simulink model "model2"  (R2023a)
settings: Solver=ode45  StartTime=0.0  StopTime=6  FixedStep=dt  MaxStep=0.001  RelTol=1e-3
values from neighbouring files (symbols this model uses):
  A = simplify(A)    [controllabilityLevel_btw.m]    (also in linearizationSS_syms.m = subs(nabla_fVec_x, args_vec, S0))
  B = simplify(B)    [controllabilityLevel_btw.m]    (also in linearizationSS_syms.m = subs(nabla_fVec_u, args_vec, S0))
  C = subs(nabla_hVec_x, args_vec, S0)    [linearizationSS_syms.m]    (also in main1_finHorLQR_OperatingPoint.m = eye(4,4); main2_finHorLQR_program_Trajectory.m = eye(4,4))
  D = subs(nabla_hVec_u, args_vec, S0)    [linearizationSS_syms.m]    (also in main1_finHorLQR_OperatingPoint.m = zeros(4,1); main2_finHorLQR_program_Trajectory.m = zeros(4,1))
  enableLinmodel = 0    [ALLINONE.m]    (also in main1_finHorLQR_OperatingPoint.m = 1; main2_finHorLQR_program_Trajectory.m)
  IC = [track_len/2, pi, 0, 0]'    [ALLINONE.m]    (also in main1_finHorLQR_OperatingPoint.m = [track_len/2;the0deg*pi/180;0;0]; main2_finHorLQR_program_Trajectory.m = [track_len/2;the0deg*pi/180;0;0])
  sat = [12, -12]    [ALLINONE.m]    (also in main1_finHorLQR_OperatingPoint.m; main2_finHorLQR_program_Trajectory.m)
settings Model: Creator=Adam  LastModifiedBy=domrazek
settings SolverCC: AlgebraicLoopSolver=TrustRegion
settings DataIOCC: ExternalInput=ind  LoadExternalInput=on  SignalLogging=off  DSMLogging=off  OutputSaveName=out  ReturnWorkspaceOutputsName=sout
settings OptimizationCC: SimCompilerOptimization=on  AccelVerboseBuild=on
settings DebuggingCC: AlgebraicLoopMsg=none  UnconnectedInputMsg=warning  UnconnectedOutputMsg=warning  UnconnectedLineMsg=warning
settings ModelReferenceCC: EnableRefExpFcnMdlSchedulingChecks=on
settings RTWCC: DLArmComputeVersion=19.05

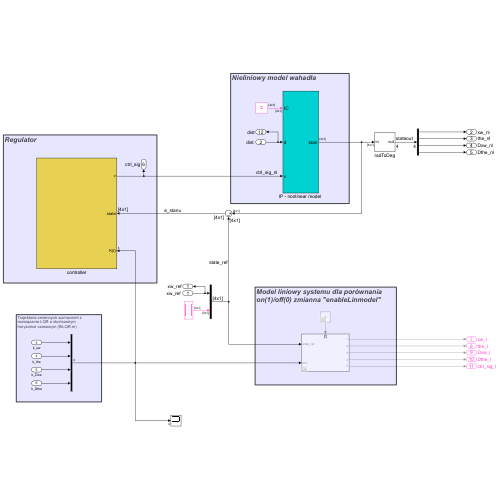
[thumbnail: Simulink's stored preview of the top-level diagram]
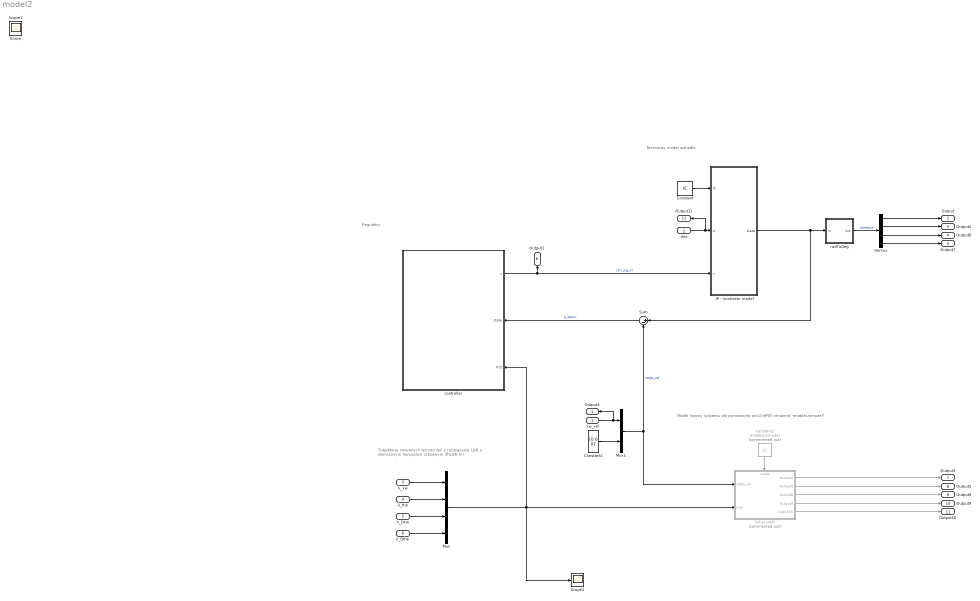
== system model2 ==
  note: Trajektoria zmiennych wzmocnień z
      | rozwiązania LQR o skończonym
      | horyzońce czasowym (fhLQR.m)
  note: Model liniowy systemu dla porównania
      | on(1)/off(0) zmianna "enableLinmodel"
  note: Nieliniowy model wahadła
  note: Regulator
  xw_ref : Inport
  dist : Inport  Port=2
  k_xw : Inport  Port=3
  k_the : Inport  Port=4
  k_Dxw : Inport  Port=5
  k_Dthe : Inport  Port=6
  Constant : Constant  Value=IC  VectorParams1D=off
  Constant1 : Constant  Value=[0 0 0]'  VectorParams1D=off
  Constant2 : Constant  Commented=on  Value=enableLinmodel
  Demux : Demux
  "IP - nonlinear model " : Subsystem  Description=Nonlinear model of inverted pendulum
      mask Display:
      | port_label('output', 1, 'stan');
      | port_label('input', 1, 'IC');
      | port_label('input', 2, 'd');
      | port_label('input', 3, 'v');
  Mux : Mux
  Mux1 : Mux  Inputs=2
  Scope2 : Scope
  Subsystem : Subsystem  Commented=on
  Sum : Sum  Inputs=|+-
  controller : Subsystem
      settings: PortSchema="{\"entries\":[{\"content\":{\"sides\":[{\"content\":{},\"type\":\"ConnectorPlacement.EquallySpacedRectSide\",\"uuid\":\"6de1dc69-5efb-4201-9eee-dce886879f47\"},{\"content\":{\"connectorIds\":[\"Out1\",\"In1\",\"In2\"],\"side\":\"RIGHT\"},\"type\":\"ConnectorPlacement.EquallySpacedRectSide\",\"uuid\":\"f5fecc05-d223-4a83-8c79-e750f1bc671b\"},{\"content\":{\"side\":\"TOP\"},\"type\":\"ConnectorPlacement.EquallySpacedRectSide\",\"uuid\":\"1fb1d94d-6570-44f6-b110-6f3978b46153\"},{\"content\":{\"side\":\"BOTTOM\"},\"type\":\"ConnectorPlacement.EquallySpacedRectSide\",\"uuid\":\"9cfdfd1f-f92b-46ce-ad17-e53ae881dd94\"}]},\"type\":\"ConnectorPlacement.EquallySpacedConnector\",\"uuid\":\"82464fa0-0bcf-47e2-bfa0-6457bd20ad21\"}],\"packageUris\":[\"http://schema.mathworks.com/mf0/Connector/R2020b\"],\"version\":\"1.0\"}"
  radToDeg : Subsystem
  Output4 : Outport  SignalName=xw_ref
  Output : Outport  Port=2  SignalName=xw_nl
  Output2 : Outport  Port=3  SignalName=the_nl
  Output6 : Outport  Port=4  SignalName=Dxw_nl
  Output7 : Outport  Port=5  SignalName=Dthe_nl
  Output1 : Outport  Port=6  SignalName=ctrl_sig
  Output3 : Outport  Port=7  SignalName=xw_l
  Output5 : Outport  Port=8  SignalName=the_l
  Output8 : Outport  Port=9  SignalName=Dxw_l
  Output9 : Outport  Port=10  SignalName=Dthe_l
  Output10 : Outport  Port=11  SignalName=ctrl_sig_l
  Output11 : Outport  Port=12  SignalName=dist
  Scope : Scope
  Scope1 : Scope
  wires:
  "IP - nonlinear model "/1(state) -> radToDeg/1(in), Sum/1
  Constant/1 -> "IP - nonlinear model "/1(IC)
  controller/1(v) -> Output1/1, "IP - nonlinear model "/3(v)  "ctrl_sig_nl"
  Sum/1 -> controller/1(state)  "e_stanu"
  dist/1 -> Output11/1, "IP - nonlinear model "/2(d)
  radToDeg/1(out) -> Demux/1  "stateout"
  Constant1/1 -> Mux1/2
  xw_ref/1 -> Output4/1, Mux1/1
  Mux1/1 -> Subsystem/1(state_ref), Sum/2  "state_ref"
  Demux/1 -> Output/1
  Demux/2 -> Output2/1
  Demux/3 -> Output6/1
  Demux/4 -> Output7/1
  Subsystem/1(Output3) -> Output3/1
  Subsystem/2(Output5) -> Output5/1
  Subsystem/3(Output8) -> Output8/1
  Subsystem/4(Output9) -> Output9/1
  Subsystem/5(Output10) -> Output10/1
  Constant2/1 -> Subsystem/Enable
  k_xw/1 -> Mux/1
  k_the/1 -> Mux/2
  k_Dxw/1 -> Mux/3
  k_Dthe/1 -> Mux/4
  Mux/1 -> Scope2/1, Subsystem/2(K(t)), controller/2(K(t))

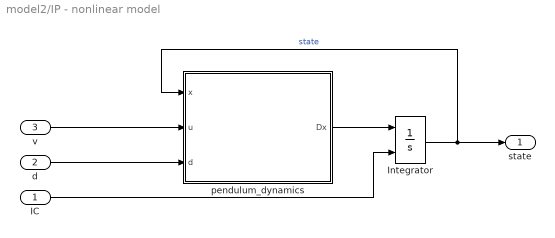
== system model2/IP - nonlinear model  ==
  IC : Inport
  d : Inport  Port=2
  v : Inport  Port=3
  Integrator : Integrator  InitialConditionSource=external
  pendulum_dynamics : MATLAB Function  TreatAsAtomicUnit=on
  state : Outport
  wires:
  Integrator/1 -> state/1, pendulum_dynamics/1(x)  "state"
  v/1 -> pendulum_dynamics/2(u)
  pendulum_dynamics/1(Dx) -> Integrator/1
  IC/1 -> Integrator/2
  d/1 -> pendulum_dynamics/3(d)

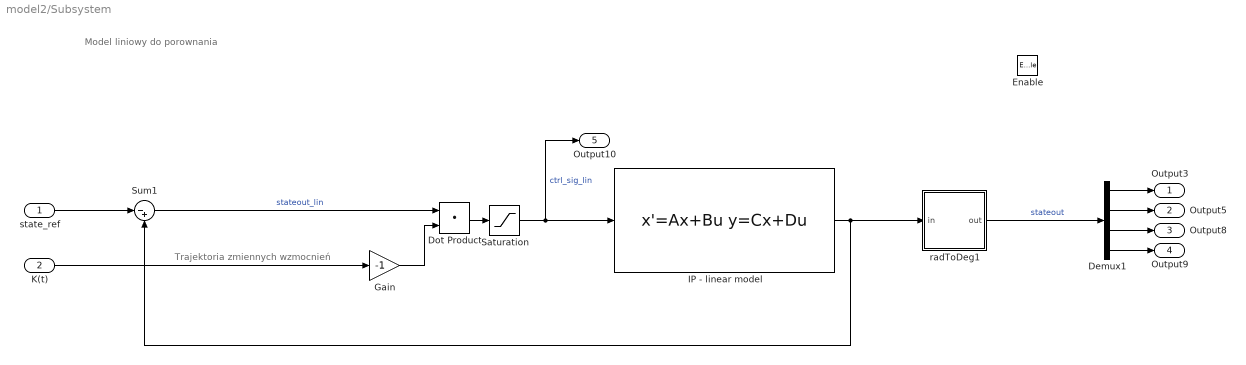
== system model2/Subsystem ==
  note: Trajektoria zmiennych wzmocnień
  note: Model liniowy do porownania
  state_ref : Inport
  K(t) : Inport  Port=2
  Enable : EnablePort
  Demux1 : Demux
  Dot Product : DotProduct  OutDataTypeStr=Inherit: Inherit via internal rule
  Gain : Gain  Gain=-1
  IP - linear model : StateSpace  A=A  B=B  C=C  D=D  InitialCondition=IC
  Saturation : Saturate  UpperLimit=sat(1)  LowerLimit=sat(2)
  Sum1 : Sum  Inputs=|-+
  radToDeg1 : Subsystem
  Output3 : Outport
  Output5 : Outport  Port=2
  Output8 : Outport  Port=3
  Output9 : Outport  Port=4
  Output10 : Outport  Port=5
  wires:
  Sum1/1 -> Dot Product/1  "stateout_lin"
  Demux1/2 -> Output5/1
  state_ref/1 -> Sum1/1
  Demux1/3 -> Output8/1
  radToDeg1/1(out) -> Demux1/1  "stateout"
  Dot Product/1 -> Saturation/1
  IP - linear model/1 -> Sum1/2, radToDeg1/1(in)
  Saturation/1 -> Output10/1, IP - linear model/1  "ctrl_sig_lin"
  Demux1/1 -> Output3/1
  Demux1/4 -> Output9/1
  K(t)/1 -> Gain/1
  Gain/1 -> Dot Product/2

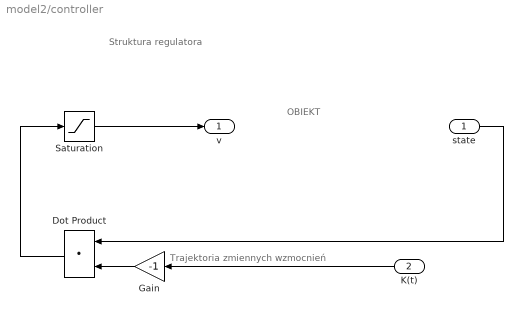
== system model2/controller ==
  note: Trajektoria zmiennych wzmocnień
  note: Struktura regulatora
  note: OBIEKT
  state : Inport
  K(t) : Inport  Port=2
  Dot Product : DotProduct  OutDataTypeStr=Inherit: Inherit via internal rule
  Gain : Gain  Gain=-1
  Saturation : Saturate  UpperLimit=sat(1)  LowerLimit=sat(2)
  v : Outport
  wires:
  Dot Product/1 -> Saturation/1
  Saturation/1 -> v/1
  state/1 -> Dot Product/1
  K(t)/1 -> Gain/1
  Gain/1 -> Dot Product/2

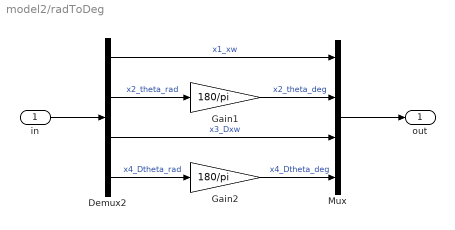
== system model2/radToDeg ==
  in : Inport
  Demux2 : Demux
  Gain1 : Gain  Gain=180/pi
  Gain2 : Gain  Gain=180/pi
  Mux : Mux
  out : Outport
  wires:
  Demux2/1 -> Mux/1  "x1_xw"
  Gain1/1 -> Mux/2  "x2_theta_deg"
  Gain2/1 -> Mux/4  "x4_Dtheta_deg"
  Demux2/2 -> Gain1/1  "x2_theta_rad"
  in/1 -> Demux2/1
  Demux2/3 -> Mux/3  "x3_Dxw"
  Demux2/4 -> Gain2/1  "x4_Dtheta_rad"
  Mux/1 -> out/1

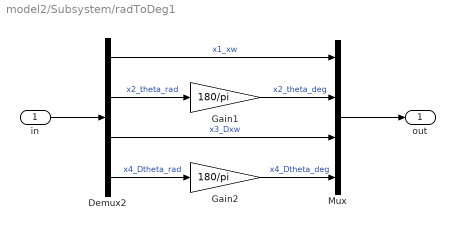
== system model2/Subsystem/radToDeg1 ==
  in : Inport
  Demux2 : Demux
  Gain1 : Gain  Gain=180/pi
  Gain2 : Gain  Gain=180/pi
  Mux : Mux
  out : Outport
  wires:
  Demux2/1 -> Mux/1  "x1_xw"
  Gain1/1 -> Mux/2  "x2_theta_deg"
  Gain2/1 -> Mux/4  "x4_Dtheta_deg"
  Demux2/2 -> Gain1/1  "x2_theta_rad"
  in/1 -> Demux2/1
  Demux2/3 -> Mux/3  "x3_Dxw"
  Demux2/4 -> Gain2/1  "x4_Dtheta_rad"
  Mux/1 -> out/1

== matlab function model2/IP - nonlinear model /pendulum_dynamics ==
  data: x input; u input; d input; Dx output; params_lepkie parameter
function Dx = dynamika_wahadla(x, u, d, params_lepkie)
% x : stan
% u : input - napięcie
%
% params scope: "parameters"
%

% State, function input: x = [x Dx theta Dtheta]'
x1 = x(1);
x2 = x(2); 
x3 = x(3);
x4 = x(4);

params_lepkie = num2cell(params_lepkie);
[M, mc, mp, Lp, Lc, g, b, gamma, mr, Mt, L, Jcm, Jt, alpha, beta] = params_lepkie{:};

% Equations for pendulum dynamics
Ff = b*x3;
Fi = alpha*u - beta*x3;
A = d*cos(x2) - Ff + L*mr*x4^2*sin(x2) + Fi;
B = d*Lc + L*g*mr*sin(x2) - gamma*x4;
DEN = Jt*Mt - (L*mr*cos(x2))^2;

ddt_x1 = x3;
ddt_x2 = x4;
ddt_x3 = (Jt*A - L*mr*cos(x2)*B) / DEN;
ddt_x4 = (Mt*B - L*mr*cos(x2)*A) / DEN;

% output (wektor kolumnowy)
Dx = [ddt_x1 ddt_x2 ddt_x3 ddt_x4]';

end
